simulink library "model_ref_lib"  (Simulink 7.9)
settings: Solver=ode45  StartTime=0.0  StopTime=10.0  RelTol=1e-3
libraries: model_ref_lib x3
settings Model: Creator=qa_user  LastModifiedBy=developer

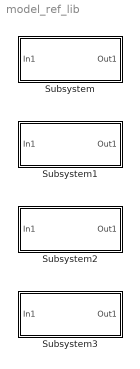
== system model_ref_lib ==
  Subsystem : Subsystem
  Subsystem1 : Subsystem
  Subsystem2 : Subsystem
  Subsystem3 : Subsystem

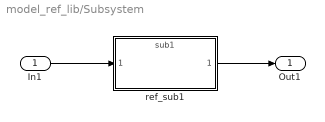
== system model_ref_lib/Subsystem ==
  In1 : Inport
  ref_sub1 : ModelReference  ModelNameDialog=sub1  ModelReferenceVersion=1.12  CopyOfModelName=sub1  DefaultDataLogging=off
  Out1 : Outport
  wires:
  In1/1 -> ref_sub1/1
  ref_sub1/1 -> Out1/1

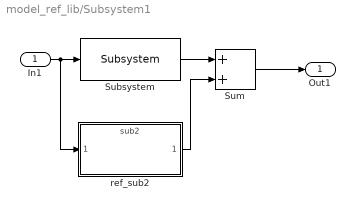
== system model_ref_lib/Subsystem1 ==
  In1 : Inport
  Subsystem : model_ref_lib/Subsystem  SystemSampleTime=-1
  Sum : Sum  mask(TL_Sum){data={'date',736211.63381096069}}
      settings: CopyFcn=if exist('tl_reset_reviewflag') == 2, tl_reset_reviewflag(gcbh); end  DeleteFcn=if exist('delete_tlblock','file')==2,delete_tlblock(gcbh);end  NameChangeFcn=if exist('rename_tlblock','file')==2,rename_tlblock(gcbh);end  OpenFcn=if exist('tl_open_blockdlg','file')==2,tl_open_blockdlg(gcbh);else,open_system(gcbh,'parameter');end
      mask Help: eval(['if exist(''tl_online_help'',''file'') == 2, tl_online_help(''Topic'',''TL_Sum''),else, web([''jar:file:///'',matlabroot,''/help/toolbox/simulink/help.jar!/slref/' lower(get_param(gcbh,'Blocktype')) '.html''], ''-helpbrowser''),end'])
      mask Display: plot([-0.05, 1.05, NaN, -0.05, 1.05],[.01, .01, NaN, .99, .99])
  ref_sub2 : ModelReference  ModelNameDialog=sub2  ModelReferenceVersion=1.15  CopyOfModelName=sub2  DefaultDataLogging=off
  Out1 : Outport
  wires:
  In1/1 -> Subsystem/1, ref_sub2/1
  Subsystem/1 -> Sum/1
  Sum/1 -> Out1/1
  ref_sub2/1 -> Sum/2

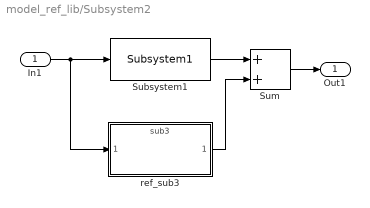
== system model_ref_lib/Subsystem2 ==
  In1 : Inport
  Subsystem1 : model_ref_lib/Subsystem1  SystemSampleTime=-1
  Sum : Sum  mask(TL_Sum){data={'date',736211.63474711811}}
      settings: CopyFcn=if exist('tl_reset_reviewflag') == 2, tl_reset_reviewflag(gcbh); end  DeleteFcn=if exist('delete_tlblock','file')==2,delete_tlblock(gcbh);end  NameChangeFcn=if exist('rename_tlblock','file')==2,rename_tlblock(gcbh);end  OpenFcn=if exist('tl_open_blockdlg','file')==2,tl_open_blockdlg(gcbh);else,open_system(gcbh,'parameter');end
      mask Help: eval(['if exist(''tl_online_help'',''file'') == 2, tl_online_help(''Topic'',''TL_Sum''),else, web([''jar:file:///'',matlabroot,''/help/toolbox/simulink/help.jar!/slref/' lower(get_param(gcbh,'Blocktype')) '.html''], ''-helpbrowser''),end'])
      mask Display: plot([-0.05, 1.05, NaN, -0.05, 1.05],[.01, .01, NaN, .99, .99])
  ref_sub3 : ModelReference  ModelNameDialog=sub3  ModelReferenceVersion=1.13  CopyOfModelName=sub3  DefaultDataLogging=off
  Out1 : Outport
  wires:
  In1/1 -> Subsystem1/1, ref_sub3/1
  Subsystem1/1 -> Sum/1
  Sum/1 -> Out1/1
  ref_sub3/1 -> Sum/2

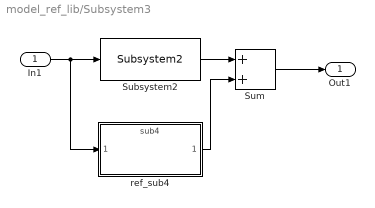
== system model_ref_lib/Subsystem3 ==
  In1 : Inport
  Subsystem2 : model_ref_lib/Subsystem2  SystemSampleTime=-1
  Sum : Sum  mask(TL_Sum){data={'date',736211.63616828702}}
      settings: CopyFcn=if exist('tl_reset_reviewflag') == 2, tl_reset_reviewflag(gcbh); end  DeleteFcn=if exist('delete_tlblock','file')==2,delete_tlblock(gcbh);end  NameChangeFcn=if exist('rename_tlblock','file')==2,rename_tlblock(gcbh);end  OpenFcn=if exist('tl_open_blockdlg','file')==2,tl_open_blockdlg(gcbh);else,open_system(gcbh,'parameter');end
      mask Help: eval(['if exist(''tl_online_help'',''file'') == 2, tl_online_help(''Topic'',''TL_Sum''),else, web([''jar:file:///'',matlabroot,''/help/toolbox/simulink/help.jar!/slref/' lower(get_param(gcbh,'Blocktype')) '.html''], ''-helpbrowser''),end'])
      mask Display: plot([-0.05, 1.05, NaN, -0.05, 1.05],[.01, .01, NaN, .99, .99])
  ref_sub4 : ModelReference  ModelNameDialog=sub4  ModelReferenceVersion=1.14  CopyOfModelName=sub4  DefaultDataLogging=off
  Out1 : Outport
  wires:
  In1/1 -> Subsystem2/1, ref_sub4/1
  Subsystem2/1 -> Sum/1
  ref_sub4/1 -> Sum/2
  Sum/1 -> Out1/1
